simulink library "fun"  (Simulink 7.0)
PreLoadFcn:
  | if exist('tl_preloadfcn','file'), tl_preloadfcn(gcs,100); end
PostLoadFcn:
  | if exist('tl_postloadfcn','file'), tl_postloadfcn(gcs,100); end
undefined symbols (not defined in the file or in its folder): KFUN_EBoostHVBattSOCMinEntry_pct, KFUN_EBoostHVBattSOCMinExit_pct
libraries: simulink x2
settings Model: TLRevision=100  Creator=pg2  LastModifiedBy=eb8

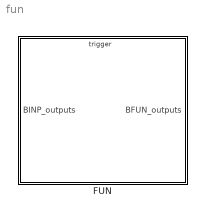
== system fun ==
  FUN : Subsystem

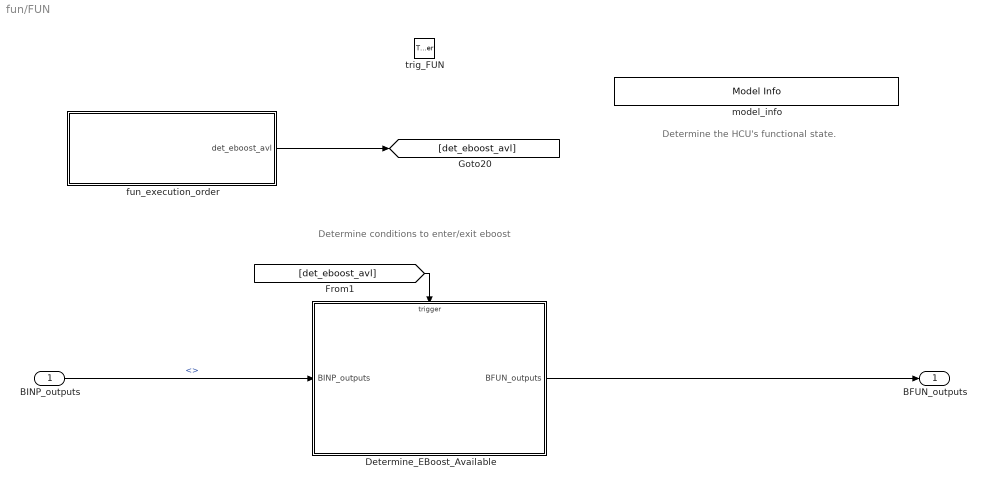
== system fun/FUN ==
  note: Determine conditions to enter/exit eboost
  note: Determine the HCU's functional state.
  BINP_outputs : Inport  UseBusObject=on  OutDataType=fixdt(1, 16)  OutScaling=2^0
      settings: BusObject=BINP_outputs
  trig_FUN : TriggerPort  TriggerType=function-call
  Determine_EBoost_Available : Subsystem
  fun_execution_order : Stateflow chart
      settings: PermitHierarchicalResolution=ParametersOnly
  model_info : simulink/Model-Wide Utilities/Model Info  SystemSampleTime=-1  InitialBlockCM=None  BlockCM=None  Frame=on  DisplayStringWithTags=$Id: fun.mdl 2 2019-09-19 09:28:50Z JuneXmas $  HorizontalTextAlignment=Center  LeftAlignmentValue=0.5  SourceBlockDiagram=tpaadd47d0_0368_43af_a7c6_f3d898c871f5  TagMaxNumber=20
  BFUN_outputs : Outport  UseBusObject=on  OutDataType=fixdt(1, 16)  OutScaling=2^0
      settings: BusObject=BFUN_outputs
  wires:
  BINP_outputs/1 -> Determine_EBoost_Available/1(BINP_outputs)  "<>"
  [det_eboost_avl] -> Determine_EBoost_Available/Trigger
  fun_execution_order/1(det_eboost_avl) -> [det_eboost_avl]
  Determine_EBoost_Available/1(BFUN_outputs) -> BFUN_outputs/1

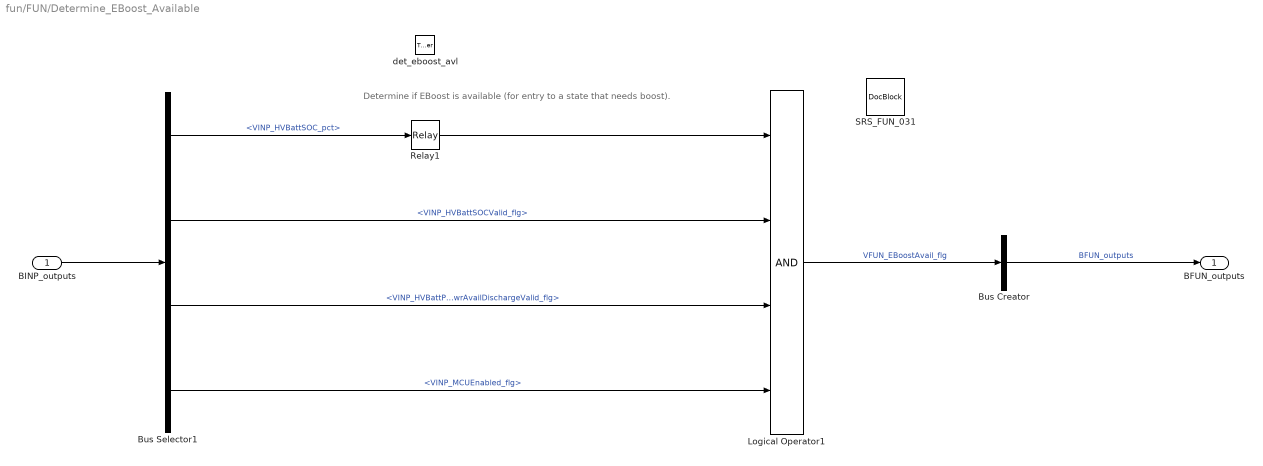
== system fun/FUN/Determine_EBoost_Available ==
  note: Determine if EBoost is available (for entry to
      | a state that needs boost).
  BINP_outputs : Inport  UseBusObject=on  OutDataType=sfix(16)  OutScaling=2^0
      settings: BusObject=BINP_outputs
  det_eboost_avl : TriggerPort  TriggerType=function-call
  Bus Creator : BusCreator  Inputs=1  UseBusObject=on
      settings: BusObject=BFUN_outputs
  Bus Selector1 : BusSelector  OutputSignals=VINP_HVBattSOC_pct,VINP_HVBattSOCValid_flg,VINP_HVBattPwrAvailDischargeValid_flg,VINP_MCUEnabled_flg
  Logical Operator1 : Logic  Inputs=4  AllPortsSameDT=off  OutDataTypeMode=boolean  LogicDataType=fixdt(0, 8)
  Relay1 : Relay  OnSwitchValue=KFUN_EBoostHVBattSOCMinEntry_pct  OffSwitchValue=KFUN_EBoostHVBattSOCMinExit_pct  OutDataType=fixdt(1, 16)  OutScaling=2^0
      settings: AttributesFormatString=%<OnSwitchValue>\n%<OffSwitchValue>
  SRS_FUN_031 : simulink/Model-Wide Utilities/DocBlock  SystemSampleTime=-1  DocumentType=Text
      content=|
      | Type your documentation here
  BFUN_outputs : Outport  UseBusObject=on  OutDataType=sfix(16)  OutScaling=2^0
      settings: BusObject=BFUN_outputs
  wires:
  Bus Creator/1 -> BFUN_outputs/1  "BFUN_outputs"
  Bus Selector1/1 -> Relay1/1  "<VINP_HVBattSOC_pct>"
  BINP_outputs/1 -> Bus Selector1/1
  Logical Operator1/1 -> Bus Creator/1  "VFUN_EBoostAvail_flg"
  Relay1/1 -> Logical Operator1/1
  Bus Selector1/2 -> Logical Operator1/2  "<VINP_HVBattSOCValid_flg>"
  Bus Selector1/3 -> Logical Operator1/3  "<VINP_HVBattPwrAvailDischargeValid_flg>"
  Bus Selector1/4 -> Logical Operator1/4  "<VINP_MCUEnabled_flg>"

== stateflow chart FUN/fun_execution_order ==
  (default) -> (junction 3)
  (junction 3) -> (junction 4) : {
      | det_eboost_avl;
      | }
  events: det_eboost_avl output FUNCTION_CALL_EVENT
